simulink model "fuel_control"  (R2020b)
settings: Solver=VariableStepAuto  StartTime=0.0  StopTime=10.0  RelTol=1e-3
values from neighbouring files (symbols this model uses):
  ego_sw = 1    [data.m]
  engine_speed = 300    [data.m]
  map_sw = 1    [data.m]
  speed_sw = 1    [data.m]
  throttle_sw = 1    [data.m]
libraries: simulink x1
settings Model: Creator=Rasika Shejul  LastModifiedBy=Rasika Shejul

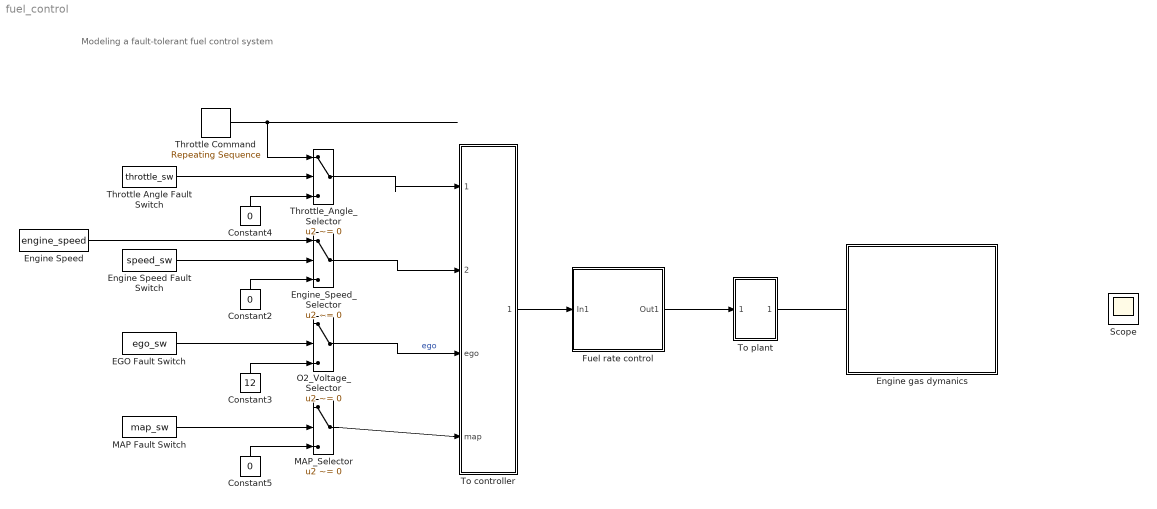
== system fuel_control ==
  note: Modeling a fault-tolerant fuel control system
  Constant2 : Constant  Value=0
  Constant3 : Constant  Value=12
  Constant4 : Constant  Value=0
  Constant5 : Constant  Value=0
  EGO Fault Switch : Constant  Value=ego_sw
  Engine Speed : Constant  Value=engine_speed  SampleTime=[0,1]
  Engine Speed Fault Switch : Constant  Value=speed_sw
  Engine gas dymanics : Subsystem
  Engine_Speed_Selector : Switch  Criteria=u2 ~= 0  Threshold=1
  Fuel rate control : Subsystem  TreatAsAtomicUnit=on
  MAP Fault Switch : Constant  Value=map_sw
  MAP_Selector : Switch  Criteria=u2 ~= 0  Threshold=1
  O2_Voltage_Selector : Switch  Criteria=u2 ~= 0  Threshold=1
  Scope : Scope
  Throttle Command : simulink/Sources/Repeating Sequence  rep_seq_t=[0 2 4]  rep_seq_y=[10 20 10]
  Throttle Angle Fault Switch : Constant  Value=throttle_sw
  Throttle_Angle_Selector : Switch  Criteria=u2 ~= 0  Threshold=1
  To controller : Subsystem
  To plant : Subsystem
  wires:
  Throttle_Angle_Selector/1 -> To controller/1(throttle)
  Engine_Speed_Selector/1 -> To controller/2(speed)
  MAP_Selector/1 -> To controller/4(map)
  To controller/1(sensors) -> Fuel rate control/1(In1)
  ? -> MAP_Selector/1
  EGO Fault Switch/1 -> O2_Voltage_Selector/2
  Constant5/1 -> MAP_Selector/3
  Throttle Command/1 -> Throttle_Angle_Selector/1
  ? -> O2_Voltage_Selector/1
  Throttle Angle Fault Switch/1 -> Throttle_Angle_Selector/2
  Engine Speed/1 -> Engine_Speed_Selector/1
  Constant2/1 -> Engine_Speed_Selector/3
  Constant3/1 -> O2_Voltage_Selector/3
  Constant4/1 -> Throttle_Angle_Selector/3
  Engine Speed Fault Switch/1 -> Engine_Speed_Selector/2
  MAP Fault Switch/1 -> MAP_Selector/2
  O2_Voltage_Selector/1 -> To controller/3(ego)  "ego"
  Fuel rate control/1(Out1) -> To plant/1(In1)
  To plant/1(Out1) -> ?

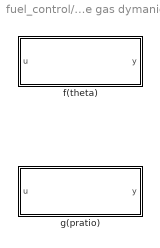
== system fuel_control/Engine gas dymanics ==
  f(theta) : MATLAB Function  TreatAsAtomicUnit=on
  g(pratio) : MATLAB Function  TreatAsAtomicUnit=on

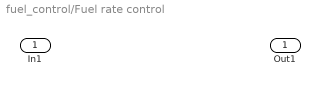
== system fuel_control/Fuel rate control ==
  In1 : Inport
  Out1 : Outport

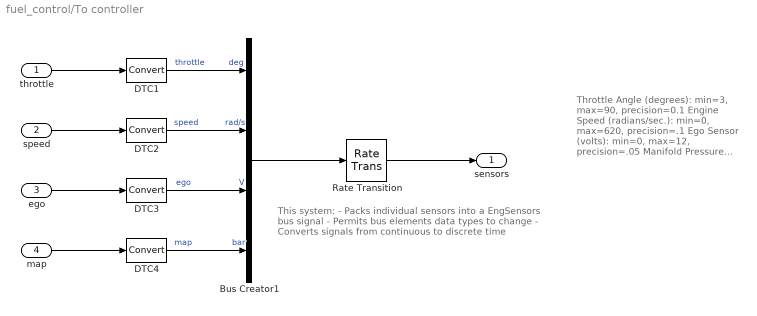
== system fuel_control/To controller ==
  note: Throttle Angle (degrees):
      | min=3, max=90, precision=0.1
      |
      | Engine Speed (radians/sec.):
      | min=0, max=620, precision=.1
      |
      | Ego Sensor (volts):
      | min=0, max=12, precision=.05
      |
      | Manifold Pressure (bar):
      | min=0.001, max=1, precision=.001
  note: This system:
      | - Packs individual sensors into a EngSensors bus signal
      | - Permits bus elements data types to change
      | - Converts signals from continuous to discrete time
  throttle : Inport
  speed : Inport  Port=2
  ego : Inport  Port=3
  map : Inport  Port=4
  Bus Creator1 : BusCreator  Inputs=4  OutDataTypeStr=Bus: EngSensors  NonVirtualBus=on
  DTC{1..4} (4 alike) : DataTypeConversion  SampleTime=[0 1]
  Rate Transition : RateTransition  OutPortSampleTime=0.01
  sensors : Outport  VectorParamsAs1DForOutWhenUnconnected=off
  wires:
  map/1 -> DTC4/1
  speed/1 -> DTC2/1
  ego/1 -> DTC3/1
  DTC2/1 -> Bus Creator1/2  "speed          rad/s"
  throttle/1 -> DTC1/1
  DTC1/1 -> Bus Creator1/1  "throttle         deg"
  DTC3/1 -> Bus Creator1/3  "ego                  V"
  Bus Creator1/1 -> Rate Transition/1
  DTC4/1 -> Bus Creator1/4  "map               bar"
  Rate Transition/1 -> sensors/1

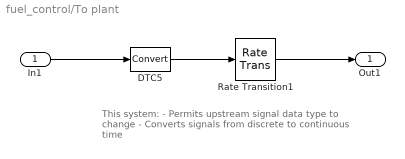
== system fuel_control/To plant ==
  note: This system:
      | - Permits upstream signal data type to change
      | - Converts signals from discrete to continuous time
  In1 : Inport
  DTC5 : DataTypeConversion
  Rate Transition1 : RateTransition  Integrity=off  InitialCondition=1.6  OutPortSampleTime=0
  Out1 : Outport  VectorParamsAs1DForOutWhenUnconnected=off
  wires:
  In1/1 -> DTC5/1
  Rate Transition1/1 -> Out1/1
  DTC5/1 -> Rate Transition1/1

== matlab function fuel_control/Engine gas dymanics/f(theta) ==
  data: u input; y output
function y = fcn(u)

y = 2.821 - 0.05231*u + 0.10299*u^2 - 0.00063*u^3;

== matlab function fuel_control/Engine gas dymanics/g(pratio) ==
  data: u input; y output
function y = fcn(u)

y = 2*sqrt(u - u^2);
